simulink model "Motor_CC_Simulink_R2017b"  (R2018a)
settings: Solver=VariableStepAuto  StartTime=0.0  StopTime=Tsim  MaxStep=1e-4  RelTol=1e-3
InitFcn:
  | Tsim = 3;
  | 
  | % Parâmetros do motor %
  | 
  | Ra = 0.6;
  | La = 0.012;
  | J = 1;
  | B = 0.1;
  | 
  | K = 1.8;
  | 
  | TC = 0;
  | TL = 10;
  | 
  | % Barramento CC %
  | 
  | Va = 30;
values from neighbouring files (symbols this model uses):
  kPWM = 1.2341    [ParameterEstimation.m]
  ktg = 0.0148    [ParameterEstimation.m]
libraries: powerlib x5, powerlib_meascontrol x1
settings Model: Creator=Daniel S. de Castro  LastModifiedBy=joaovitor

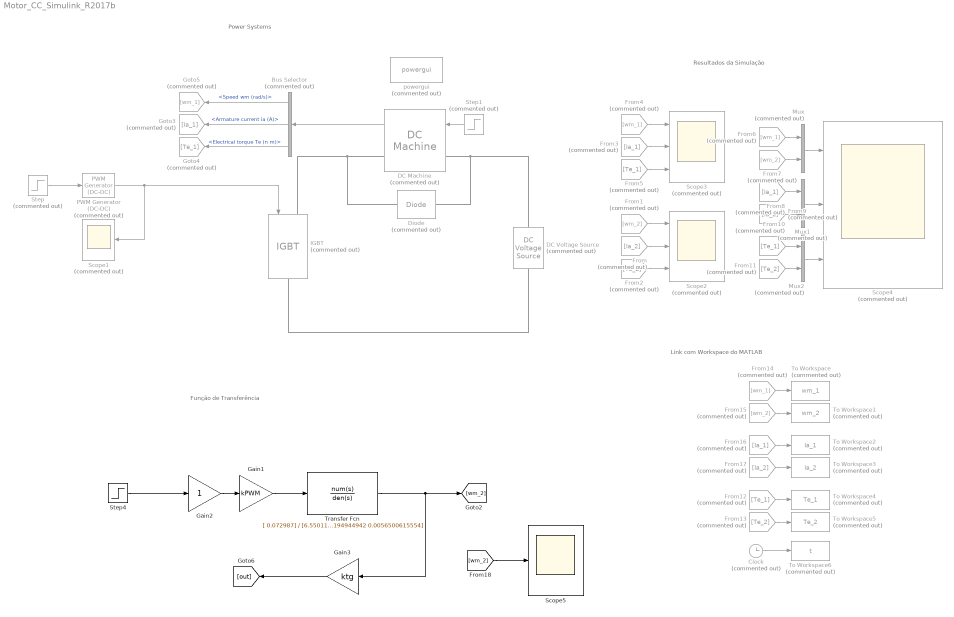
== system Motor_CC_Simulink_R2017b ==
  note: Resultados da Simulação
  note: Power Systems
  note: Função de Transferência
  note: Link com Workspace do MATLAB
  Bus Selector : BusSelector  Commented=on  OutputSignals=Speed wm (rad/s),Armature current ia (A),Electrical torque Te (n m)
  Clock : Clock  Commented=on
  DC Machine : powerlib/Machines/DC Machine  Commented=on  PresetModel=No  MechanicalLoad=Torque TL  FieldType=Permanent magnet  ShowDetailedParameters=on  MeasurementBus=off  RLa=[Ra La]  RLf="[ 240  120]"  Laf=1.8  MachineConstant=Torque constant (N.m/A)  Ke=1.8  Kt=K  J=J  Bm=B  Tf=TC  w0=0  Ifinit=1  TsPowergui=0  TsBlock=-1
  DC Voltage Source : powerlib/Electrical Sources/DC Voltage Source  Commented=on  Amplitude=Va  Measurements=None
  Diode : powerlib/Power Electronics/Diode  Commented=on  Ron=0  Lon=0  Vf=0  IC=0  UseSnubber=0  Rs=inf  Cs=inf  Measurements=off
  From : From  Commented=on  GotoTag=Ia_2
  From1 : From  Commented=on  GotoTag=wm_2
  From10 : From  Commented=on  GotoTag=Te_1
  From11 : From  Commented=on  GotoTag=Te_2
  From12 : From  Commented=on  GotoTag=Te_1
  From13 : From  Commented=on  GotoTag=Te_2
  From14 : From  Commented=on  GotoTag=wm_1
  From15 : From  Commented=on  GotoTag=wm_2
  From16 : From  Commented=on  GotoTag=Ia_1
  From17 : From  Commented=on  GotoTag=Ia_2
  From2 : From  Commented=on  GotoTag=Te_2
  From3 : From  Commented=on  GotoTag=Ia_1
  From4 : From  Commented=on  GotoTag=wm_1
  From5 : From  Commented=on  GotoTag=Te_1
  From6 : From  Commented=on  GotoTag=wm_1
  From7 : From  Commented=on  GotoTag=wm_2
  From8 : From  Commented=on  GotoTag=Ia_1
  From9 : From  Commented=on  GotoTag=Ia_2
  Gain1 : Gain  Gain=kPWM
  Gain2 : Gain
  Gain3 : Gain  Gain=ktg
  Goto3 : Goto  Commented=on  GotoTag=Ia_1
  Goto4 : Goto  Commented=on  GotoTag=Te_1
  Goto5 : Goto  Commented=on  GotoTag=wm_1
  IGBT : powerlib/Power Electronics/IGBT  Commented=on  Ron=0  Lon=0  Vf=0  Tf=1e-6  Tt=2e-6  IC=0  Rs=inf  Cs=inf  Measurements=off
  Mux : Mux  Commented=on  Inputs=2
  Mux1 : Mux  Commented=on  Inputs=2
  Mux2 : Mux  Commented=on  Inputs=2
  PWM Generator (DC-DC) : powerlib_meascontrol/Pulse & Signal Generators/PWM Generator (DC-DC)  Commented=on  Fsw=1000  Ts=0
  Scope1 : Scope  Commented=on
  Scope2 : Scope  Commented=on  NumInputPorts=3
  Scope3 : Scope  Commented=on  NumInputPorts=3
  Scope4 : Scope  Commented=on  NumInputPorts=3
  Scope5 : Scope
  Step : Step  Commented=on  After=10  SampleTime=0
  Step1 : Step  Commented=on  Time=2  After=TL  SampleTime=0
  Step4 : Step  After=10  SampleTime=0
  To Workspace : ToWorkspace  Commented=on  VariableName=wm_1  SampleTime=-1
  To Workspace1 : ToWorkspace  Commented=on  VariableName=wm_2  SampleTime=-1
  To Workspace2 : ToWorkspace  Commented=on  VariableName=Ia_1  SampleTime=-1
  To Workspace3 : ToWorkspace  Commented=on  VariableName=Ia_2  SampleTime=-1
  To Workspace4 : ToWorkspace  Commented=on  VariableName=Te_1  SampleTime=-1
  To Workspace5 : ToWorkspace  Commented=on  VariableName=Te_2  SampleTime=-1
  To Workspace6 : ToWorkspace  Commented=on  VariableName=t  SampleTime=-1
  Transfer Fcn : TransferFcn  Numerator=[ 0.072987]  Denominator=[6.55011645e-09 0.0001087194944942 0.0056500615554]
  powergui : powerlib/powergui  Priority=1  Commented=on  SimulationMode=Continuous  SampleTime=50e-6  frequency=60  Iterations=50  frequencyindice=0  Pbase=100e6  ErrMax=1e-4  UnitsV=kV  UnitsW=MW  buscounter=0  FunctionMessages=off  echomessages=off  EnableUseOfTLC=off  CurrentSourceSwitches=off  DisableSnubberDevices=off  DisableRonSwitches=off  DisableVfSwitches=off  DisplayEquations=off  SolverType=Tustin/Backward Euler (TBE)  Interpol=off  ExternalGateDelay=off  methode=off  Ts=100  x0status=blocks  SPID=on  SwTol=0  HookPort=off  RestoreLinks=warning  ResistiveCurrentMeasurement=off  Frange=[0:2:500]  Ylog=off  Xlog=on  ShowGrid=off  save=off  variable=ZData  structure=0  ZoomFFT=off  StartTime=0.0  cycles=1  DisplayStyle=1  fundamental=60  FreqAxis=off  MaxFrequency=1000  frequencyindicesteady=1  RmsSteady=1  display=off
  wires:
  PWM Generator (DC-DC)/1 -> Scope1/1, IGBT/1
  DC Machine/1 -> Bus Selector/1
  Bus Selector/1 -> Goto5/1  "<Speed wm (rad/s)>"
  Bus Selector/2 -> Goto3/1  "<Armature current ia (A)>"
  Step1/1 -> DC Machine/1
  Bus Selector/3 -> Goto4/1  "<Electrical torque Te (n m)>"
  Step/1 -> PWM Generator (DC-DC)/1
  Transfer Fcn/1 -> [wm_2], Gain3/1
  From/1 -> Scope2/2
  From1/1 -> Scope2/1
  From2/1 -> Scope2/3
  From4/1 -> Scope3/1
  From5/1 -> Scope3/3
  From3/1 -> Scope3/2
  Mux/1 -> Scope4/1
  From6/1 -> Mux/1
  From7/1 -> Mux/2
  Mux1/1 -> Scope4/2
  Mux2/1 -> Scope4/3
  From8/1 -> Mux1/1
  From9/1 -> Mux1/2
  From10/1 -> Mux2/1
  From11/1 -> Mux2/2
  From12/1 -> To Workspace4/1
  From17/1 -> To Workspace3/1
  From14/1 -> To Workspace/1
  From16/1 -> To Workspace2/1
  From15/1 -> To Workspace1/1
  From13/1 -> To Workspace5/1
  Clock/1 -> To Workspace6/1
  Step4/1 -> Gain2/1
  Gain3/1 -> [out]
  [wm_2] -> Scope5/1
  Gain2/1 -> Gain1/1
  Gain1/1 -> Transfer Fcn/1
  connections:
  DC Voltage Source/RConn1 -- Diode/RConn1 -- DC Machine/LConn1
  DC Machine/RConn1 -- IGBT/LConn1 -- Diode/LConn1
  IGBT/RConn1 -- DC Voltage Source/LConn1
